simulink model "simpleW"  (R2016b)
settings: Solver=VariableStepAuto  StartTime=0.0  StopTime=10.0  RelTol=1e-3
libraries: powerlib_meascontrol x1
settings Model: Creator=Roozbeh  LastModifiedBy=Roozbeh

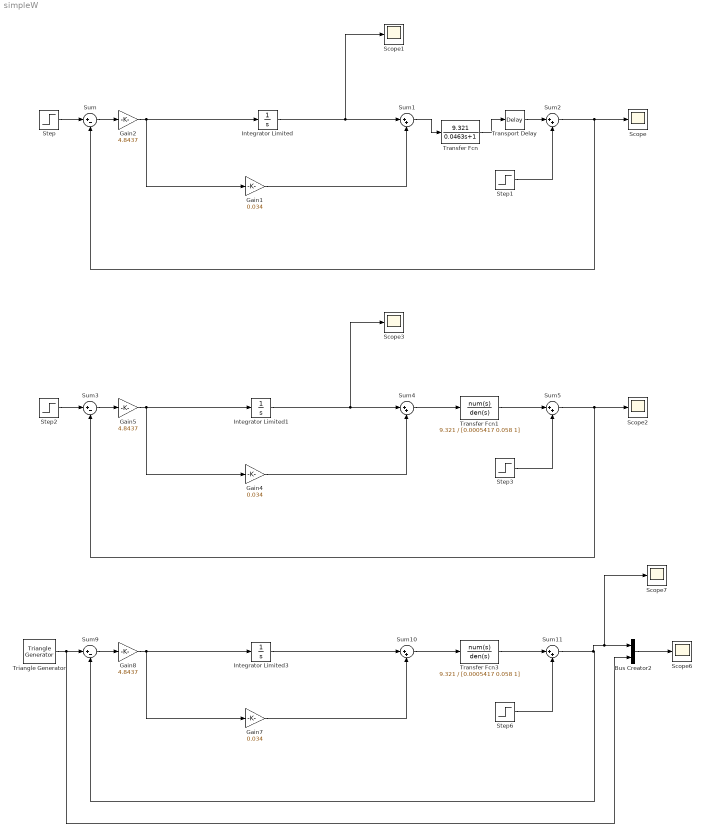
== system simpleW ==
  Bus Creator2 : BusCreator  Inputs=2
  Gain1 : Gain  Gain=0.034
  Gain2 : Gain  Gain=4.8437
  Gain4 : Gain  Gain=0.034
  Gain5 : Gain  Gain=4.8437
  Gain7 : Gain  Gain=0.034
  Gain8 : Gain  Gain=4.8437
  Integrator Limited : Integrator  LimitOutput=on  UpperSaturationLimit=0.5  LowerSaturationLimit=-0.5
  Integrator Limited1 : Integrator  LimitOutput=on  UpperSaturationLimit=0.5  LowerSaturationLimit=-0.5
  Integrator Limited3 : Integrator  LimitOutput=on  UpperSaturationLimit=0.5  LowerSaturationLimit=-0.5
  Scope{,1..3,6..7} (6 alike) : Scope
  Step : Step  SampleTime=0
  Step1 : Step  Time=1.02  After=0  SampleTime=0
  Step2 : Step  SampleTime=0
  Step3 : Step  Time=20  After=5  SampleTime=0
  Step6 : Step  Time=20  After=0  SampleTime=0
  Sum : Sum  Inputs=|+-
  Sum{1..2,4..5,10..11} (6 alike) : Sum  Inputs=|++
  Sum3 : Sum  Inputs=|+-
  Sum9 : Sum  Inputs=|+-
  Transfer Fcn : TransferFcn  Numerator=9.321  Denominator=[0.0463 1]
  Transfer Fcn1 : TransferFcn  Numerator=9.321  Denominator=[0.0005417 0.058 1]
  Transfer Fcn3 : TransferFcn  Numerator=9.321  Denominator=[0.0005417 0.058 1]
  Transport Delay : TransportDelay  DelayTime=0.0117
  Triangle Generator : powerlib_meascontrol/Pulse & Signal Generators/Triangle Generator  Freq=1  Phase=90  Ts=0
  wires:
  Step/1 -> Sum/1
  Sum1/1 -> Transfer Fcn/1
  Sum/1 -> Gain2/1
  Gain2/1 -> Integrator Limited/1, Gain1/1
  Gain1/1 -> Sum1/2
  Sum2/1 -> Sum/2, Scope/1
  Step1/1 -> Sum2/2
  Transfer Fcn/1 -> Transport Delay/1
  Transport Delay/1 -> Sum2/1
  Sum4/1 -> Transfer Fcn1/1
  Sum3/1 -> Gain5/1
  Gain5/1 -> Integrator Limited1/1, Gain4/1
  Gain4/1 -> Sum4/2
  Sum5/1 -> Scope2/1, Sum3/2
  Step3/1 -> Sum5/2
  Transfer Fcn1/1 -> Sum5/1
  Integrator Limited/1 -> Scope1/1, Sum1/1
  Integrator Limited1/1 -> Scope3/1, Sum4/1
  Step2/1 -> Sum3/1
  Sum10/1 -> Transfer Fcn3/1
  Sum9/1 -> Gain8/1
  Gain8/1 -> Gain7/1, Integrator Limited3/1
  Gain7/1 -> Sum10/2
  Sum11/1 -> Scope7/1, Bus Creator2/1, Sum9/2
  Step6/1 -> Sum11/2
  Transfer Fcn3/1 -> Sum11/1
  Integrator Limited3/1 -> Sum10/1
  Triangle Generator/1 -> Bus Creator2/2, Sum9/1
  Bus Creator2/1 -> Scope6/1
